simulink model "lab6"  (R2016a)
settings: Solver=ode45  StartTime=0.0  StopTime=50  MaxStep=0.04  RelTol=1e-3
libraries: simulink x1
settings Model: Creator=ms36124  LastModifiedBy=ms36124

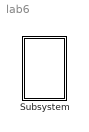
== system lab6 ==
  Subsystem : Subsystem  mask{g=9.81, k1=2, k2=1, m1=1, m2=1.4, R=0.001, l1=1, l2=2, f1=80, f2=150, M=1, r0=2, fi0=90}

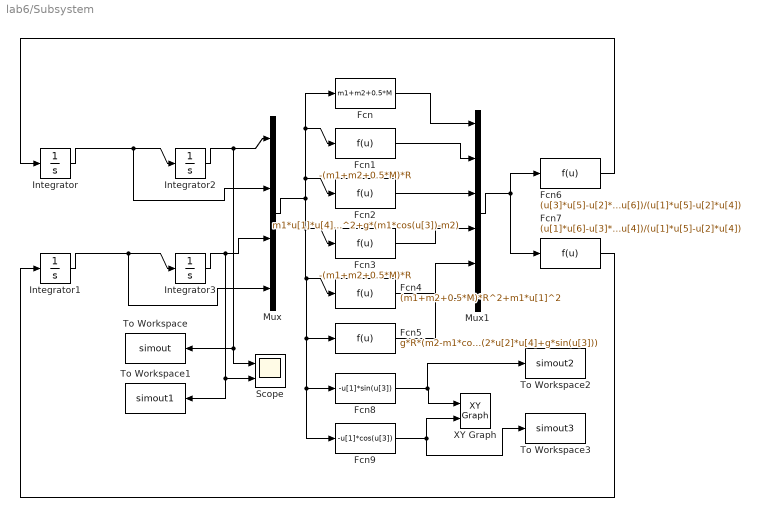
== system lab6/Subsystem ==
  Fcn : Fcn  Expr=m1+m2+0.5*M
  Fcn1 : Fcn  Expr=-(m1+m2+0.5*M)*R
  Fcn2 : Fcn  Expr=m1*u[1]*u[4]^2+g*(m1*cos(u[3])-m2)
  Fcn3 : Fcn  Expr=-(m1+m2+0.5*M)*R
  Fcn4 : Fcn  Expr=(m1+m2+0.5*M)*R^2+m1*u[1]^2
  Fcn5 : Fcn  Expr=g*R*(m2-m1*cos(u[3]))-m1*u[1]*(2*u[2]*u[4]+g*sin(u[3]))
  Fcn6 : Fcn  Expr=(u[3]*u[5]-u[2]*u[6])/(u[1]*u[5]-u[2]*u[4])
  Fcn7 : Fcn  Expr=(u[1]*u[6]-u[3]*u[4])/(u[1]*u[5]-u[2]*u[4])
  Fcn8 : Fcn  Expr=-u[1]*sin(u[3])
  Fcn9 : Fcn  Expr=-u[1]*cos(u[3])
  Integrator : Integrator
  Integrator1 : Integrator
  Integrator2 : Integrator  InitialCondition=r0
  Integrator3 : Integrator  InitialCondition=fi0*pi/180
  Mux : Mux
  Mux1 : Mux  Inputs=6
  Scope : Scope  NumInputPorts=2
  To Workspace : ToWorkspace  VariableName=simout  SaveFormat=Timeseries  SampleTime=-1
  To Workspace1 : ToWorkspace  VariableName=simout1  SaveFormat=Timeseries  SampleTime=-1
  To Workspace2 : ToWorkspace  VariableName=simout2  SaveFormat=Timeseries  SampleTime=-1
  To Workspace3 : ToWorkspace  VariableName=simout3  SaveFormat=Timeseries  SampleTime=-1
  XY Graph : simulink/Sinks/XY Graph  xmin=-4  xmax=4  ymin=-4  ymax=4  st=-1
  wires:
  Mux/1 -> Fcn2/1, Fcn1/1, Fcn/1, Fcn9/1, Fcn8/1, Fcn5/1, Fcn4/1, Fcn3/1
  Fcn/1 -> Mux1/1
  Fcn7/1 -> Integrator1/1
  Mux1/1 -> Fcn7/1, Fcn6/1
  Integrator3/1 -> To Workspace1/1, Scope/2, Mux/3
  Integrator1/1 -> Mux/4, Integrator3/1
  Fcn2/1 -> Mux1/3
  Integrator2/1 -> To Workspace/1, Scope/1, Mux/1
  Fcn5/1 -> Mux1/6
  Integrator/1 -> Mux/2, Integrator2/1
  Fcn1/1 -> Mux1/2
  Fcn6/1 -> Integrator/1
  Fcn3/1 -> Mux1/4
  Fcn4/1 -> Mux1/5
  Fcn8/1 -> To Workspace2/1, XY Graph/1
  Fcn9/1 -> To Workspace3/1, XY Graph/2
